simulink model "Copy_of_AB_Final_of_MPC_Bandwidth_Result"  (R2022b)
settings: Solver=FixedStepDiscrete  StartTime=0.0  StopTime=Inf  FixedStep=100e-6  RelTol=1e-3  EnableMultiTasking=on
undefined symbols (not defined in the file): C28x, CPU1, CPU2, CurrentBypassValue, DiscIntNeverNeededParam, Down, GPTRIP1SEL, TZ1, Up
libraries: c2802xlib x31, simulink x22, dspstat3 x17, dspsigops x9, c2837xDlib x6, c280xlib x5, PID_Lib x2, c2000lib x1, spsAlphaBetaZerotoabcLib x1, spsAlphaBetaZerotodq0Lib x1
(part 2 of 8)

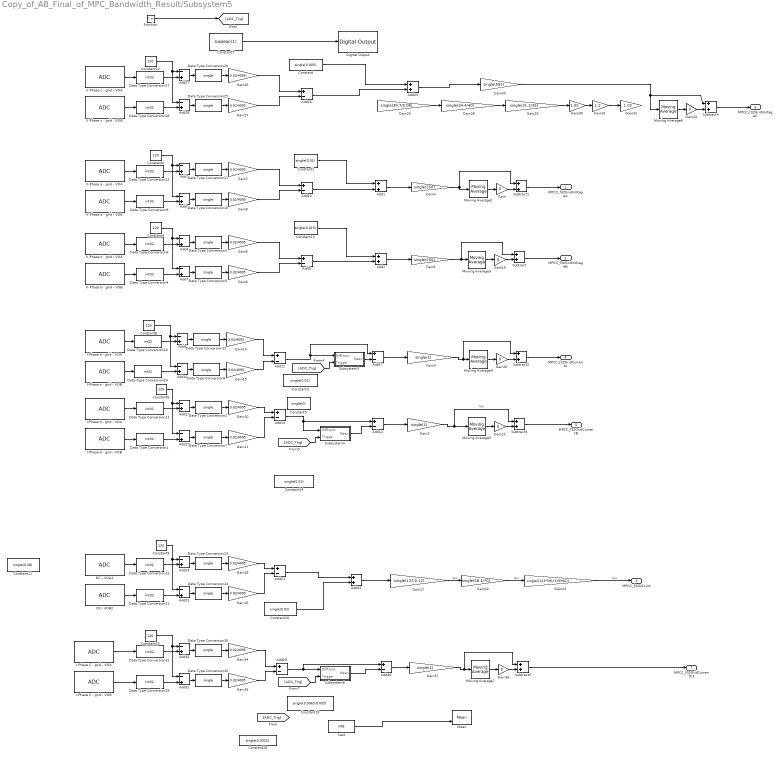
== system Copy_of_AB_Final_of_MPC_Bandwidth_Result/Subsystem5 ==
  function : TriggerPort  TriggerType=function-call  VariantControl=(inherit)  ShowOutputPort=on  OutputDataType=int8
  Add{1..2,22,25} (4 alike) : Sum  AccumDataTypeStr=single  OutDataTypeStr=single
  Add{5,10,12..14,17,21,26,29..30} (10 alike) : Sum  Inputs=+-  AccumDataTypeStr=single  OutDataTypeStr=single
  Add{3..4,6..7,9,11,15,18,23..24,27..28,31..32} (14 alike) : Sum  Inputs=-+  AccumDataTypeStr=single  OutDataTypeStr=single
  Cast : DataTypeConversion  OutDataTypeStr=int8  SaturateOnIntegerOverflow=off  RndMeth=Floor
  Constant : Constant  Value=single(0.005)
  Constant1 : Constant  Value=single(0.01)
  Constant10 : Constant  Value=single(0.02)
  Constant11 : Constant  Value=single(0.28)
  Constant{2,4,6,8..9,12,15} (7 alike) : Constant  Value=120  OutDataTypeStr=single
  Constant13 : Constant  Value=single(0.015)
  Constant14 : Constant  Value=single(0.01)
  Constant18 : Constant  Value=single(0.0025)
  Constant19 : Constant  Value=single(0.0065-0.005)
  Constant3 : Constant  Value=single(0.01)
  Constant5 : Constant  Value=single(0)
  Constant7 : Constant  Value=boolean(1)
  DC - VOA2 : c2802xlib/ADC  blkParamProc=C2000_Type4  ADCModule=C  samplingMode=Single sample mode  ADCResolution=12-bit (Single-ended input)  useSOC1=SOC0  useSOC2=SOC0_SOC1  SOCAcquisitionWindow=22  SOCTriggerSource=ePWM1_ADCSOCA  SOCInterruptTrigger=No ADCINT  Ts=-1  dType=uint16  postInterrupt=off  interruptSel=ADCINT1  ADCINTContinuous=on  endma=off  chdma=1  conv1=ADCINA0  conv2=ADCINA0 and ADCINB0  conv1_Type4=ADCIN5  conv2_Type4=ADCIN0 and ADCIN1
  DC- VOB2 : c2802xlib/ADC  blkParamProc=C2000_Type4  ADCModule=B  samplingMode=Single sample mode  ADCResolution=12-bit (Single-ended input)  useSOC1=SOC3  useSOC2=SOC0_SOC1  SOCAcquisitionWindow=22  SOCTriggerSource=ePWM1_ADCSOCA  SOCInterruptTrigger=No ADCINT  Ts=-1  dType=uint16  postInterrupt=off  interruptSel=ADCINT2  ADCINTContinuous=on  endma=off  chdma=1  conv1=ADCINA0  conv2=ADCINA0 and ADCINB0  conv1_Type4=ADCIN5  conv2_Type4=ADCIN2 and ADCIN3
  Data Type Conversion{1,4,6,9,12..14,16,21..22,27..29,31} (14 alike) : DataTypeConversion  OutDataTypeStr=int32  ConvertRealWorld=Stored Integer (SI)  SaturateOnIntegerOverflow=off  RndMeth=Floor
  Data Type Conversion{2..3,5,7..8,10..11,15,23..26,30,32} (14 alike) : DataTypeConversion  OutDataTypeStr=single  SaturateOnIntegerOverflow=off  RndMeth=Floor
  Digital Output : c2837xDlib/Digital Output  GPIO_Number=GPIO32~GPIO39  GPIO_Bit0=on  GPIO_BIT0_Toggle=on  GPIO_Bit1=off  GPIO_BIT1_Toggle=off  GPIO_Bit2=off  GPIO_BIT2_Toggle=off  GPIO_Bit3=off  GPIO_BIT3_Toggle=off  GPIO_Bit4=off  GPIO_BIT4_Toggle=off  GPIO_Bit5=off  GPIO_BIT5_Toggle=off  GPIO_Bit6=off  GPIO_BIT6_Toggle=off  GPIO_Bit7=off  GPIO_BIT7_Toggle=off
  Gain{,19..21,24,36} (6 alike) : Gain  Gain=0
  Gain1 : Gain  Gain=single(250)
  Gain{5..7,9..11,14..16,18,26..27,34..35} (14 alike) : Gain  Gain=3.02/4095  ParamDataTypeStr=single  OutDataTypeStr=single
  Gain17 : Gain  Gain=single(137/0.22)
  Gain2 : Gain  Gain=single(1)
  Gain22 : Gain  Gain=single(58.4/70)
  Gain23 : Gain  Gain=single((123*59)/(135*60))
  Gain25 : Gain  Gain=single(30.7/0.06)
  Gain28 : Gain  Gain=single(34.4/40)
  Gain29 : Gain  Gain=single(31.2/35)
  Gain3 : Gain  Gain=single(1)
  Gain30 : Gain  Gain=1.05
  Gain31 : Gain  Gain=1.2
  Gain32 : Gain  Gain=1.02
  Gain33 : Gain  Gain=single(505)
  Gain37 : Gain  Gain=single(1)
  Gain4 : Gain  Gain=single(250)
  I-Phase C - grid - VOA : c2802xlib/ADC  blkParamProc=C2000_Type4  ADCModule=A  samplingMode=Single sample mode  ADCResolution=12-bit (Single-ended input)  useSOC1=SOC15  useSOC2=SOC0_SOC1  SOCAcquisitionWindow=22  SOCTriggerSource=ePWM1_ADCSOCA  SOCInterruptTrigger=No ADCINT  Ts=-1  dType=uint16  postInterrupt=off  interruptSel=ADCINT1  ADCINTContinuous=on  endma=off  chdma=1  conv1=ADCINA0  conv2=ADCINA0 and ADCINB0  conv1_Type4=ADCIN15  conv2_Type4=ADCIN0 and ADCIN1
  I-Phase C - grid - VOB : c2802xlib/ADC  blkParamProc=C2000_Type4  ADCModule=A  samplingMode=Single sample mode  ADCResolution=12-bit (Single-ended input)  useSOC1=SOC10  useSOC2=SOC0_SOC1  SOCAcquisitionWindow=22  SOCTriggerSource=ePWM1_ADCSOCA  SOCInterruptTrigger=No ADCINT  Ts=-1  dType=uint16  postInterrupt=off  interruptSel=ADCINT2  ADCINTContinuous=on  endma=off  chdma=1  conv1=ADCINA0  conv2=ADCINA0 and ADCINB0  conv1_Type4=ADCIN14  conv2_Type4=ADCIN2 and ADCIN3
  I-Phase a - grid - VOA : c2802xlib/ADC  blkParamProc=C2000_Type4  ADCModule=A  samplingMode=Single sample mode  ADCResolution=12-bit (Single-ended input)  useSOC1=SOC0  useSOC2=SOC0_SOC1  SOCAcquisitionWindow=22  SOCTriggerSource=ePWM1_ADCSOCA  SOCInterruptTrigger=No ADCINT  Ts=-1  dType=uint16  postInterrupt=on  interruptSel=ADCINT1  ADCINTContinuous=on  endma=off  chdma=1  conv1=ADCINA0  conv2=ADCINA0 and ADCINB0  conv1_Type4=ADCIN4  conv2_Type4=ADCIN0 and ADCIN1
  I-Phase a - grid - VOB : c2802xlib/ADC  blkParamProc=C2000_Type4  ADCModule=B  samplingMode=Single sample mode  ADCResolution=12-bit (Single-ended input)  useSOC1=SOC1  useSOC2=SOC0_SOC1  SOCAcquisitionWindow=22  SOCTriggerSource=ePWM1_ADCSOCA  SOCInterruptTrigger=No ADCINT  Ts=-1  dType=uint16  postInterrupt=off  interruptSel=ADCINT2  ADCINTContinuous=on  endma=off  chdma=1  conv1=ADCINA0  conv2=ADCINA0 and ADCINB0  conv1_Type4=ADCIN4  conv2_Type4=ADCIN2 and ADCIN3
  I-Phase b - grid - VOA : c2802xlib/ADC  blkParamProc=C2000_Type4  ADCModule=C  samplingMode=Single sample mode  ADCResolution=12-bit (Single-ended input)  useSOC1=SOC12  useSOC2=SOC0_SOC1  SOCAcquisitionWindow=22  SOCTriggerSource=ePWM1_ADCSOCA  SOCInterruptTrigger=No ADCINT  Ts=-1  dType=uint16  postInterrupt=off  interruptSel=ADCINT1  ADCINTContinuous=on  endma=off  chdma=1  conv1=ADCINA0  conv2=ADCINA0 and ADCINB0  conv1_Type4=ADCIN4  conv2_Type4=ADCIN0 and ADCIN1
  I-Phase b - grid - VOB : c2802xlib/ADC  blkParamProc=C2000_Type4  ADCModule=A  samplingMode=Single sample mode  ADCResolution=12-bit (Single-ended input)  useSOC1=SOC3  useSOC2=SOC0_SOC1  SOCAcquisitionWindow=22  SOCTriggerSource=ePWM1_ADCSOCA  SOCInterruptTrigger=No ADCINT  Ts=-1  dType=uint16  postInterrupt=off  interruptSel=ADCINT2  ADCINTContinuous=on  endma=off  chdma=1  conv1=ADCINA0  conv2=ADCINA0 and ADCINB0  conv1_Type4=ADCIN5  conv2_Type4=ADCIN2 and ADCIN3
  Mean : dspstat3/Mean  run=on  InputProcessing=Columns as channels (frame based)  reset_popup=Rising edge  directionMode=Each column  dimension=1  roiEnable=off  roiType=Rectangles  roiPortion=Entire ROI  roiOutput=Individual statistics for each ROI  roiFlag=off  roundingMode=Floor  overflowMode=off  outputDataTypeStr=Inherit: Same as accumulator  outputMin=[]  outputMax=[]  outputLastDataTypeStr=Inherit: Same as accumulator
  Moving Average{1,3..7} (6 alike) : dspstat3/Moving Average  Method=Exponential weighting  ForgettingFactorPort=off  SpecifyWindowLength=on  WindowLength=4  OverlapLength=3  AllowArbitraryInputLength=off  ForgettingFactor=0.99  SimulateUsing=Code generation
  Subsystem3 : Subsystem
  Subsystem4 : Subsystem
  Subsystem6 : Subsystem
  Subtract{,1..5} (6 alike) : Sum
  V-Phase a - grid - VOA : c2802xlib/ADC  blkParamProc=C2000_Type4  ADCModule=C  samplingMode=Single sample mode  ADCResolution=12-bit (Single-ended input)  useSOC1=SOC4  useSOC2=SOC0_SOC1  SOCAcquisitionWindow=22  SOCTriggerSource=ePWM1_ADCSOCA  SOCInterruptTrigger=No ADCINT  Ts=-1  dType=uint16  postInterrupt=off  interruptSel=ADCINT1  ADCINTContinuous=on  endma=off  chdma=1  conv1=ADCINA0  conv2=ADCINA0 and ADCINB0  conv1_Type4=ADCIN3  conv2_Type4=ADCIN0 and ADCIN1
  V-Phase a - grid - VOB : c2802xlib/ADC  blkParamProc=C2000_Type4  ADCModule=B  samplingMode=Single sample mode  ADCResolution=12-bit (Single-ended input)  useSOC1=SOC5  useSOC2=SOC0_SOC1  SOCAcquisitionWindow=22  SOCTriggerSource=ePWM1_ADCSOCA  SOCInterruptTrigger=No ADCINT  Ts=-1  dType=uint16  postInterrupt=off  interruptSel=ADCINT2  ADCINTContinuous=on  endma=off  chdma=1  conv1=ADCINA0  conv2=ADCINA0 and ADCINB0  conv1_Type4=ADCIN3  conv2_Type4=ADCIN2 and ADCIN3
  V-Phase b - grid - VOA : c2802xlib/ADC  blkParamProc=C2000_Type4  ADCModule=A  samplingMode=Single sample mode  ADCResolution=12-bit (Single-ended input)  useSOC1=SOC6  useSOC2=SOC0_SOC1  SOCAcquisitionWindow=22  SOCTriggerSource=ePWM1_ADCSOCA  SOCInterruptTrigger=No ADCINT  Ts=-1  dType=uint16  postInterrupt=off  interruptSel=ADCINT1  ADCINTContinuous=on  endma=off  chdma=1  conv1=ADCINA0  conv2=ADCINA0 and ADCINB0  conv1_Type4=ADCIN3  conv2_Type4=ADCIN0 and ADCIN1
  V-Phase b - grid - VOB : c2802xlib/ADC  blkParamProc=C2000_Type4  ADCModule=C  samplingMode=Single sample mode  ADCResolution=12-bit (Single-ended input)  useSOC1=SOC7  useSOC2=SOC0_SOC1  SOCAcquisitionWindow=22  SOCTriggerSource=ePWM1_ADCSOCA  SOCInterruptTrigger=No ADCINT  Ts=-1  dType=uint16  postInterrupt=off  interruptSel=ADCINT2  ADCINTContinuous=on  endma=off  chdma=1  conv1=ADCINA0  conv2=ADCINA0 and ADCINB0  conv1_Type4=ADCIN2  conv2_Type4=ADCIN2 and ADCIN3
  V-Phase c - grid - VOA : c2802xlib/ADC  blkParamProc=C2000_Type4  ADCModule=B  samplingMode=Single sample mode  ADCResolution=12-bit (Single-ended input)  useSOC1=SOC0  useSOC2=SOC0_SOC1  SOCAcquisitionWindow=22  SOCTriggerSource=ePWM1_ADCSOCA  SOCInterruptTrigger=No ADCINT  Ts=-1  dType=uint16  postInterrupt=off  interruptSel=ADCINT1  ADCINTContinuous=on  endma=off  chdma=1  conv1=ADCINA0  conv2=ADCINA0 and ADCINB0  conv1_Type4=ADCIN2  conv2_Type4=ADCIN0 and ADCIN1
  V-Phase c - grid - VOB : c2802xlib/ADC  blkParamProc=C2000_Type4  ADCModule=A  samplingMode=Single sample mode  ADCResolution=12-bit (Single-ended input)  useSOC1=SOC1  useSOC2=SOC0_SOC1  SOCAcquisitionWindow=22  SOCTriggerSource=ePWM1_ADCSOCA  SOCInterruptTrigger=No ADCINT  Ts=-1  dType=uint16  postInterrupt=off  interruptSel=ADCINT2  ADCINTContinuous=on  endma=off  chdma=1  conv1=ADCINA0  conv2=ADCINA0 and ADCINB0  conv1_Type4=ADCIN2  conv2_Type4=ADCIN2 and ADCIN3
  MPCC_f32GridVoltageA : Outport
  MPCC_f32GridVoltageB : Outport  Port=2
  MPCC_f32DCLink : Outport  Port=3
  MPCC_f32GridCurrentA : Outport  Port=4
  MPCC_f32GridCurrentB : Outport  Port=5
  MPCC_f32GridVoltageC : Outport  Port=6
  MPCC_f32GridCurrentC3 : Outport  Port=7
  wires:
  Gain5/1 -> Add5/1
  Data Type Conversion5/1 -> Gain5/1
  Gain1/1 -> Subtract/1, Moving Average3/1
  Add9/1 -> Data Type Conversion10/1
  V-Phase a - grid - VOB/1 -> Data Type Conversion9/1
  Data Type Conversion9/1 -> Add9/2
  Gain7/1 -> Add10/1
  Data Type Conversion10/1 -> Gain9/1
  Data Type Conversion12/1 -> Add3/2
  Add7/1 -> Data Type Conversion3/1
  Data Type Conversion4/1 -> Add7/2
  Data Type Conversion6/1 -> Add4/2
  Gain9/1 -> Add10/2
  V-Phase b - grid - VOB/1 -> Data Type Conversion4/1
  V-Phase b - grid - VOA/1 -> Data Type Conversion6/1
  Add4/1 -> Data Type Conversion5/1
  Add3/1 -> Data Type Conversion11/1
  Data Type Conversion3/1 -> Gain6/1
  Gain6/1 -> Add5/2
  Constant4/1 -> Add7/1, Add4/1
  V-Phase a - grid - VOA/1 -> Data Type Conversion12/1
  Constant2/1 -> Add9/1, Add3/1
  Data Type Conversion11/1 -> Gain7/1
  Add1/1 -> Gain4/1
  Add2/1 -> Gain1/1
  I-Phase b - grid - VOA/1 -> Data Type Conversion13/1
  Data Type Conversion15/1 -> Gain14/1
  Data Type Conversion8/1 -> Gain15/1
  Data Type Conversion14/1 -> Add18/2
  Gain15/1 -> Add12/2
  Data Type Conversion13/1 -> Add11/2
  Data Type Conversion16/1 -> Add6/2
  Gain14/1 -> Add12/1
  Add6/1 -> Data Type Conversion15/1
  Gain10/1 -> Add13/1
  Add18/1 -> Data Type Conversion8/1
  I-Phase a - grid - VOA/1 -> Data Type Conversion16/1
  Gain2/1 -> Subtract3/1, Moving Average5/1  "Iau"
  Data Type Conversion2/1 -> Gain10/1
  Constant6/1 -> Add15/1, Add11/1
  I-Phase b - grid - VOB/1 -> Data Type Conversion1/1
  Data Type Conversion1/1 -> Add15/2
  Gain11/1 -> Add13/2
  Add17/1 -> Gain3/1
  Add11/1 -> Data Type Conversion2/1
  Constant8/1 -> Add18/1, Add6/1
  I-Phase a - grid - VOB/1 -> Data Type Conversion14/1
  Data Type Conversion7/1 -> Gain11/1
  Add15/1 -> Data Type Conversion7/1
  Subtract/1 -> MPCC_f32GridVoltageB/1
  Moving Average3/1 -> Gain19/1
  Moving Average1/1 -> Gain/1
  Gain4/1 -> Subtract1/1, Moving Average1/1
  Subtract1/1 -> MPCC_f32GridVoltageA/1
  Moving Average4/1 -> Gain20/1
  Gain3/1 -> Subtract2/1, Moving Average4/1
  Moving Average5/1 -> Gain21/1
  Data Type Conversion22/1 -> Add24/2
  DC- VOB2/1 -> Data Type Conversion21/1
  Data Type Conversion21/1 -> Add23/2
  Data Type Conversion23/1 -> Gain18/1
  DC - VOA2/1 -> Data Type Conversion22/1
  Add24/1 -> Data Type Conversion23/1
  Constant9/1 -> Add23/1, Add24/1
  Gain16/1 -> Add21/2
  Add23/1 -> Data Type Conversion24/1
  Data Type Conversion24/1 -> Gain16/1
  Gain18/1 -> Add21/1
  Gain/1 -> Subtract1/2
  Gain19/1 -> Subtract/2
  Gain20/1 -> Subtract2/2
  Gain21/1 -> Subtract3/2
  Gain17/1 -> Gain22/1  "Iau"
  Subtract2/1 -> MPCC_f32GridCurrentA/1
  Subtract3/1 -> MPCC_f32GridCurrentB/1
  Gain22/1 -> Gain23/1  "Iau"
  V-Phase c - grid - VOB/1 -> Data Type Conversion28/1
  Gain26/1 -> Add26/1
  Data Type Conversion25/1 -> Gain27/1
  V-Phase c - grid - VOA/1 -> Data Type Conversion27/1
  Subtract4/1 -> MPCC_f32GridVoltageC/1
  Data Type Conversion26/1 -> Gain26/1
  Data Type Conversion27/1 -> Add27/2
  Moving Average6/1 -> Gain24/1
  Data Type Conversion28/1 -> Add28/2
  Gain27/1 -> Add26/2
  Add28/1 -> Data Type Conversion25/1
  Constant12/1 -> Add28/1, Add27/1
  Add27/1 -> Data Type Conversion26/1
  Gain25/1 -> Gain28/1
  Gain24/1 -> Subtract4/2
  Gain28/1 -> Gain29/1
  Gain29/1 -> Gain30/1
  Gain30/1 -> Gain31/1
  Gain31/1 -> Gain32/1
  Gain33/1 -> Subtract4/1, Moving Average6/1
  Add31/1 -> Data Type Conversion32/1
  Data Type Conversion32/1 -> Gain35/1
  Data Type Conversion31/1 -> Add32/2
  Gain34/1 -> Add29/1
  Constant15/1 -> Add31/1, Add32/1
  Gain35/1 -> Add29/2
  Subtract5/1 -> MPCC_f32GridCurrentC3/1
  Gain36/1 -> Subtract5/2
  Data Type Conversion30/1 -> Gain34/1
  Data Type Conversion29/1 -> Add31/2
  I-Phase C - grid - VOB/1 -> Data Type Conversion29/1
  I-Phase C - grid - VOA/1 -> Data Type Conversion31/1
  Gain37/1 -> Subtract5/1, Moving Average7/1
  Add32/1 -> Data Type Conversion30/1
  Add30/1 -> Gain37/1
  Moving Average7/1 -> Gain36/1
  Add22/1 -> Gain17/1
  Constant7/1 -> Digital Output/1
  Add14/1 -> Gain2/1
  function/1 -> [ADC_Trig]
  Cast/1 -> Mean/2
  Add25/1 -> Gain33/1
  [ADC_Trig] -> Subsystem3/2(Trigger)
  Add12/1 -> Add17/1, Subsystem3/1(DiffInput)
  Subsystem3/1(Mean) -> Add17/2
  [ADC_Trig] -> Subsystem4/2(Trigger)
  Add13/1 -> Add14/1, Subsystem4/1(DiffInput)
  Subsystem4/1(Mean) -> Add14/2
  [ADC_Trig] -> Subsystem6/2(Trigger)
  Add29/1 -> Add30/1, Subsystem6/1(DiffInput)
  Subsystem6/1(Mean) -> Add30/2
  Constant/1 -> Add25/1
  Add26/1 -> Add25/2
  Constant1/1 -> Add1/1
  Add10/1 -> Add1/2
  Constant13/1 -> Add2/1
  Add5/1 -> Add2/2
  Gain23/1 -> MPCC_f32DCLink/1  "Iau"
  Add21/1 -> Add22/1
  Constant10/1 -> Add22/2

== system Copy_of_AB_Final_of_MPC_Bandwidth_Result/Voltage_Loop ==
  PI_f32DCLinkVoltageRef : Inport
  PI_f32DCLinkVoltage : Inport  Port=2
  PI_f32DCLink : Inport  Port=3
  VoltageLoop_FC : TriggerPort  TriggerType=function-call  VariantControl=(inherit)  SampleTime=-1
      settings: AttributesFormatString=|
      | %<StatesWhenEnabling>
      | %<SampleTime>
  Add : Sum  Inputs=+-
  Cast To Single : DataTypeConversion  OutDataTypeStr=single  SaturateOnIntegerOverflow=off  RndMeth=Floor
  Cast To Single1 : DataTypeConversion  OutDataTypeStr=single  SaturateOnIntegerOverflow=off  RndMeth=Floor
  Cast To Single3 : DataTypeConversion  OutDataTypeStr=single  SaturateOnIntegerOverflow=off  RndMeth=Floor
  Constant : Constant  Commented=on  Value=single(0.2)
  Constant1 : Constant  Commented=on  Value=single(10)
  Constant10 : Constant  Value=single(2.5)
  Constant11 : Constant  Value=single(0.1)
  Constant12 : Constant  Value=single(0.8685252)
  Constant13 : Constant  Value=single(0.01955)
  Constant2 : Constant  Value=single(7/7)
  Constant3 : Constant  Value=boolean(1)
  Constant4 : Constant  Value=boolean(0)
  Constant5 : Constant  Value=boolean(1)
  Constant6 : Constant  Value=single(0.2)
  Constant7 : Constant  Value=single(0)
  Constant8 : Constant  Commented=on  Value=CurrentBypassValue
  Constant9 : Constant  Value=single(10)
  Gain : Gain  Gain=-1
  Gain1 : Gain  Gain=single(7)
  Gain2 : Gain  Gain=1/300
  Gain3 : Gain  Gain=1/300
  Mux2 : Mux  Inputs=3
  PI : PID_Lib/PI  SystemSampleTime=-1  VariantActivationTime=update diagram  Latency=0  AutoFrameSizeCalculation=off
  Scope : Scope
  Step : Step  Time=30  Before=-0.5  After=-1.5
  Step1 : Step  Time=30  Before=200  After=300
  Subsystem5 : Subsystem  Commented=through
  Switch : Switch  Criteria=u2 ~= 0  SaturateOnIntegerOverflow=off  InputSameDT=off
  Terminator{,1..4} (5 alike) : Terminator
  PI_f32DGridCurrentReference : Outport
  MPCC_f32DCLinkFiltered : Outport  Port=2
  MPCC_f32DCLinkref : Outport  Port=3
  wires:
  Constant2/1 -> Gain/1, PI/4
  Gain/1 -> PI/5
  Constant3/1 -> PI/6
  Constant4/1 -> PI/7
  PI/2 -> Terminator/1
  PI/3 -> Terminator1/1
  PI/4 -> Terminator2/1
  PI/5 -> Terminator3/1
  Constant5/1 -> Switch/2
  PI/1 -> Switch/1, Scope/1
  Switch/1 -> Cast To Single/1
  Cast To Single1/1 -> Gain2/1
  Cast To Single/1 -> Gain1/1
  Cast To Single3/1 -> Gain3/1, MPCC_f32DCLinkref/1
  PI_f32DCLinkVoltage/1 -> Subsystem5/1(MPCC_f32DCLink)
  Subsystem5/1(MPCC_f32DCLinkFiltered) -> MPCC_f32DCLinkFiltered/1, Cast To Single1/1
  Constant7/1 -> PI/8
  Step/1 -> Switch/3
  Add/1 -> Mux2/1, PI/1
  Gain1/1 -> Mux2/2, PI_f32DGridCurrentReference/1
  Gain3/1 -> Add/1
  Gain2/1 -> Add/2
  PI_f32DCLink/1 -> Mux2/3
  Mux2/1 -> Terminator4/1
  PI_f32DCLinkVoltageRef/1 -> Cast To Single3/1
  Constant6/1 -> PI/2
  Constant9/1 -> PI/3

== system Copy_of_AB_Final_of_MPC_Bandwidth_Result/Subsystem1/ABCtoDQO ==
  PI_f32GridCurrentA : Inport
  PI_f32GridCurrentB : Inport  Port=2
  PI_f32GridCurrentC : Inport  Port=3
  PI_f32GridVoltageA : Inport  Port=4
  PI_f32GridVoltageB : Inport  Port=5
  PI_f32GridVoltageC : Inport  Port=6
  PI_f32ElectricalAngle : Inport  Port=7
  MPCC_f32AngularFrequency : Inport  Port=8
  ABCtoDQOCurrent : Subsystem  Commented=on
  ABCtoDQOVoltage : Subsystem  Commented=on
  Cast To Single : DataTypeConversion  OutDataTypeStr=single  SaturateOnIntegerOverflow=off  RndMeth=Floor
  Cast To Single1 : DataTypeConversion  OutDataTypeStr=single  SaturateOnIntegerOverflow=off  RndMeth=Floor
  Constant : Constant
  Gain1 : Gain  Gain=single(100e-6)
  Ground : Ground
  abc_dq : Subsystem
  abc_dq1 : Subsystem
  abc_dq4 : Subsystem
  PI_f32DGridCurrent : Outport
  PI_f32QGridCurrent : Outport  Port=2
  PI_f32OGridCurrent : Outport  Port=3
  PI_f32DGridVoltage : Outport  Port=4
  PI_f32QGridVoltage : Outport  Port=5
  PI_f32OGridVoltage : Outport  Port=6
  PI_f32DGridVoltage1 : Outport  Port=7
  PI_f32QGridVoltage1 : Outport  Port=8
  wires:
  abc_dq/1(Id) -> Cast To Single/1
  abc_dq/2(Iq) -> Cast To Single1/1
  PI_f32ElectricalAngle/1 -> [PI_f32ElectricalAngle]
  [PI_f32ElectricalAngle] -> abc_dq/1(theta)
  Ground/1 -> PI_f32OGridCurrent/1, PI_f32OGridVoltage/1
  abc_dq1/2(Iq) -> PI_f32QGridVoltage/1
  [PI_f32ElectricalAngle] -> abc_dq1/1(theta)
  abc_dq1/1(Id) -> PI_f32DGridVoltage/1
  PI_f32GridCurrentC/1 -> abc_dq/4(c)
  PI_f32GridCurrentB/1 -> abc_dq/3(b)
  PI_f32GridCurrentA/1 -> abc_dq/2(a)
  PI_f32GridVoltageA/1 -> abc_dq4/2(a), abc_dq1/2(a)
  PI_f32GridVoltageB/1 -> abc_dq1/3(b), abc_dq4/3(b)
  PI_f32GridVoltageC/1 -> abc_dq1/4(c), abc_dq4/4(c)
  Cast To Single/1 -> PI_f32DGridCurrent/1
  Cast To Single1/1 -> PI_f32QGridCurrent/1
  MPCC_f32AngularFrequency/1 -> [MPCC_f32AngularFrequency]
  Gain1/1 -> abc_dq4/1(theta)
  Constant/1 -> abc_dq4/5(c1)
  [MPCC_f32AngularFrequency] -> Gain1/1
  abc_dq4/1(Id) -> PI_f32DGridVoltage1/1
  abc_dq4/2(Iq) -> PI_f32QGridVoltage1/1

== system Copy_of_AB_Final_of_MPC_Bandwidth_Result/Subsystem1/AlphaBetaDutiesCalculation ==
  MPCC_f32DVoltageReference : Inport
  MPCC_f32QVoltageReference : Inport  Port=2
  MPCC_f32ElectricalAngle_K_1 : Inport  Port=3
  MPCC_f32DCLinkVoltage : Inport  Port=4
  AlphaBetaVoltageReferenceCalculation : Subsystem
  DutiesCalculation : Subsystem
  MPCC_f32AlphaVoltageReference : Outport
  MPCC_f32BetaVoltageReference : Outport  Port=2
  MPCC_f32Duty_Sector1 : Outport  Port=3
  MPCC_f32Duty_Sector2 : Outport  Port=4
  MPCC_f32Duty_Sector3 : Outport  Port=5
  MPCC_f32Duty_Sector4 : Outport  Port=6
  MPCC_f32Duty_Sector5 : Outport  Port=7
  MPCC_f32Duty_Sector6 : Outport  Port=8
  wires:
  MPCC_f32ElectricalAngle_K_1/1 -> AlphaBetaVoltageReferenceCalculation/3(MPCC_f32ElectricalAngle_K_1)
  AlphaBetaVoltageReferenceCalculation/1(MPCC_f32AlphaVoltageReference) -> MPCC_f32AlphaVoltageReference/1
  AlphaBetaVoltageReferenceCalculation/2(MPCC_f32BetaVoltageReference) -> MPCC_f32BetaVoltageReference/1
  DutiesCalculation/1(MPCC_f32Duty_Sector1) -> MPCC_f32Duty_Sector1/1
  DutiesCalculation/2(MPCC_f32Duty_Sector2) -> MPCC_f32Duty_Sector2/1
  DutiesCalculation/3(MPCC_f32Duty_Sector3) -> MPCC_f32Duty_Sector3/1
  DutiesCalculation/4(MPCC_f32Duty_Sector4) -> MPCC_f32Duty_Sector4/1
  DutiesCalculation/6(MPCC_f32Duty_Sector6) -> MPCC_f32Duty_Sector6/1
  DutiesCalculation/5(MPCC_f32Duty_Sector5) -> MPCC_f32Duty_Sector5/1
  MPCC_f32DCLinkVoltage/1 -> DutiesCalculation/3(MPCC_f32DCLinkVoltage)
  [MPCC_f32AlphaVoltageReference] -> DutiesCalculation/1(MPCC_f32AlphaVoltageReference)
  [MPCC_f32BetaVoltageReference] -> DutiesCalculation/2(MPCC_f32BetaVoltageReference)
  MPCC_f32DVoltageReference/1 -> [MPCC_f32AlphaVoltageReference]
  MPCC_f32QVoltageReference/1 -> [MPCC_f32BetaVoltageReference]

== system Copy_of_AB_Final_of_MPC_Bandwidth_Result/Subsystem1/AlphaBetaVoltageReferenceCalculation ==
  MPCC_f32DVoltageReference : Inport
  MPCC_f32QVoltageReference : Inport  Port=2
  MPCC_f32ElectricalAngle_K_1 : Inport  Port=3
  Add : Sum  Inputs=+-
  Add1 : Sum
  Product{,1..3} (4 alike) : Product
  Sin : Trigonometry  Operator=cos
  Sin1 : Trigonometry
  Sin2 : Trigonometry
  Sin3 : Trigonometry  Operator=cos
  MPCC_f32AlphaVoltageReference : Outport
  MPCC_f32BetaVoltageReference : Outport  Port=2
  wires:
  Sin2/1 -> Product2/1
  [MPCC_f32QVoltageReference] -> Product3/2
  Sin1/1 -> Product1/1
  Sin3/1 -> Product3/1
  Product/1 -> Add/1
  [MPCC_f32DVoltageReference] -> Product2/2
  [MPCC_f32ElectricalAngle_K_1] -> Sin2/1
  [MPCC_f32QVoltageReference] -> Product1/2
  Add1/1 -> MPCC_f32BetaVoltageReference/1
  Product2/1 -> Add1/1
  Product3/1 -> Add1/2
  [MPCC_f32ElectricalAngle_K_1] -> Sin3/1
  MPCC_f32DVoltageReference/1 -> [MPCC_f32DVoltageReference]
  Add/1 -> MPCC_f32AlphaVoltageReference/1
  [MPCC_f32ElectricalAngle_K_1] -> Sin/1
  [MPCC_f32DVoltageReference] -> Product/2
  MPCC_f32QVoltageReference/1 -> [MPCC_f32QVoltageReference]
  Product1/1 -> Add/2
  Sin/1 -> Product/1
  [MPCC_f32ElectricalAngle_K_1] -> Sin1/1
  MPCC_f32ElectricalAngle_K_1/1 -> [MPCC_f32ElectricalAngle_K_1]

== system Copy_of_AB_Final_of_MPC_Bandwidth_Result/Subsystem1/CodeGeneration ==
  Input : Inport
  Add : Sum  Inputs=+-  OutDataTypeStr=Inherit: Same as first input
  Demux2 : Demux  Outputs=2
  Index Vector : MultiPortSwitch  Inputs=1  SaturateOnIntegerOverflow=off  InputSameDT=off
  SCI Transmit : c280xlib/SCI Transmit  sciModule=A  dataHead=''  dataTail=''  blockingMode=on  outputStatus=off
  While Iterator : WhileIterator  MaxIters=-1  WhileBlockType=do-while  ShowIterationPort=on  OutputDataType=int16
  wires:
  While Iterator/1 -> Add/2, Index Vector/1
  Demux2/1 -> Index Vector/2
  Index Vector/1 -> SCI Transmit/1
  Add/1 -> While Iterator/1
  Demux2/2 -> Add/1
  Input/1 -> Demux2/1

== system Copy_of_AB_Final_of_MPC_Bandwidth_Result/Subsystem1/CodeGeneration1 ==
  Input : Inport
  Add : Sum  Inputs=+-  OutDataTypeStr=Inherit: Same as first input
  Demux2 : Demux  Outputs=2
  Index Vector : MultiPortSwitch  Inputs=1  SaturateOnIntegerOverflow=off  InputSameDT=off
  SCI Transmit : c280xlib/SCI Transmit  sciModule=A  dataHead=''  dataTail=''  blockingMode=on  outputStatus=off
  While Iterator : WhileIterator  MaxIters=-1  WhileBlockType=do-while  ShowIterationPort=on  OutputDataType=int16
  wires:
  While Iterator/1 -> Add/2, Index Vector/1
  Demux2/1 -> Index Vector/2
  Index Vector/1 -> SCI Transmit/1
  Add/1 -> While Iterator/1
  Demux2/2 -> Add/1
  Input/1 -> Demux2/1

== system Copy_of_AB_Final_of_MPC_Bandwidth_Result/Subsystem1/Data ==
  Data : Inport
  Data_width : Inport  Port=2
  Action Port : ActionPort  ActionPortLabel=else
  Mux : Mux  Inputs=2
  Start : Constant  Value=hex2dec('0000')  OutDataTypeStr=uint16
  Data_out : Outport  VectorParamsAs1DForOutWhenUnconnected=off
  Iteration : Outport  Port=2  VectorParamsAs1DForOutWhenUnconnected=off
  wires:
  Start/1 -> Mux/2
  Mux/1 -> Data_out/1
  Data/1 -> Mux/1
  Data_width/1 -> Iteration/1

== system Copy_of_AB_Final_of_MPC_Bandwidth_Result/Subsystem1/Data1 ==
  Data : Inport
  Data_width : Inport  Port=2
  Action Port : ActionPort  ActionPortLabel=else
  Mux : Mux  Inputs=2
  Start : Constant  Value=hex2dec('0000')  OutDataTypeStr=uint16
  Data_out : Outport  VectorParamsAs1DForOutWhenUnconnected=off
  Iteration : Outport  Port=2  VectorParamsAs1DForOutWhenUnconnected=off
  wires:
  Start/1 -> Mux/2
  Mux/1 -> Data_out/1
  Data/1 -> Mux/1
  Data_width/1 -> Iteration/1

== system Copy_of_AB_Final_of_MPC_Bandwidth_Result/Subsystem1/Data_Conditioning ==
  In1 : Inport
  Data Type Conversion3 : DataTypeConversion  OutDataTypeStr=uint16  ConvertRealWorld=Stored Integer (SI)  SaturateOnIntegerOverflow=off  RndMeth=Floor
  Out1 : Outport  VectorParamsAs1DForOutWhenUnconnected=off
  wires:
  Data Type Conversion3/1 -> Out1/1
  In1/1 -> Data Type Conversion3/1

== system Copy_of_AB_Final_of_MPC_Bandwidth_Result/Subsystem1/Data_Conditioning1 ==
  In1 : Inport
  Data Type Conversion3 : DataTypeConversion  OutDataTypeStr=uint16  ConvertRealWorld=Stored Integer (SI)  SaturateOnIntegerOverflow=off  RndMeth=Floor
  Out1 : Outport  VectorParamsAs1DForOutWhenUnconnected=off
  wires:
  Data Type Conversion3/1 -> Out1/1
  In1/1 -> Data Type Conversion3/1

== system Copy_of_AB_Final_of_MPC_Bandwidth_Result/Subsystem1/End ==
  Data : Inport
  Data_width : Inport  Port=2
  Action Port : ActionPort  ActionPortLabel=elseif(u1 == 599)
  Bias : Bias  Bias=1  SaturateOnIntegerOverflow=off
  Mux : Mux  Inputs=2
  Start : Constant  Value=hex2dec('4545')  OutDataTypeStr=uint16
  Data_out : Outport  VectorParamsAs1DForOutWhenUnconnected=off
  Iteration : Outport  Port=2  VectorParamsAs1DForOutWhenUnconnected=off
  wires:
  Mux/1 -> Data_out/1
  Data_width/1 -> Bias/1
  Start/1 -> Mux/2
  Bias/1 -> Iteration/1
  Data/1 -> Mux/1

== system Copy_of_AB_Final_of_MPC_Bandwidth_Result/Subsystem1/End1 ==
  Data : Inport
  Data_width : Inport  Port=2
  Action Port : ActionPort  ActionPortLabel=elseif(u1 == 599)
  Bias : Bias  Bias=1  SaturateOnIntegerOverflow=off
  Mux : Mux  Inputs=2
  Start : Constant  Value=hex2dec('4545')  OutDataTypeStr=uint16
  Data_out : Outport  VectorParamsAs1DForOutWhenUnconnected=off
  Iteration : Outport  Port=2  VectorParamsAs1DForOutWhenUnconnected=off
  wires:
  Mux/1 -> Data_out/1
  Data_width/1 -> Bias/1
  Start/1 -> Mux/2
  Bias/1 -> Iteration/1
  Data/1 -> Mux/1

== system Copy_of_AB_Final_of_MPC_Bandwidth_Result/Subsystem1/GridCurrentFirstPrediction ==
  MPCC_f32Predictionterm_A : Inport
  MPCC_f32Predictionterm_B : Inport  Port=2
  MPCC_f32Predictionterm_C : Inport  Port=3
  MPCC_f32DGridCurrent : Inport  Port=4
  MPCC_f32QGridCurrent : Inport  Port=5
  MPCC_f32DGridVoltage : Inport  Port=6
  MPCC_f32QGridVoltage : Inport  Port=7
  MPCC_f32DConvVoltage : Inport  Port=8
  MPCC_f32QConvVoltage : Inport  Port=9
  PredictedIdGridCurrentCalculation : Subsystem
  PredictedIqGridCurrentCalculation : Subsystem
  MPCC_f32DGridCurrent_K_1 : Outport
  MPCC_f32QGridCurrent_K_1 : Outport  Port=2
  wires:
  MPCC_f32DGridVoltage/1 -> [MPCC_f32DGridVoltage]
  MPCC_f32Predictionterm_A/1 -> [MPCC_f32Predictionterm_A]
  MPCC_f32QGridVoltage/1 -> [MPCC_f32QGridVoltage]
  MPCC_f32Predictionterm_C/1 -> [MPCC_f32Predictionterm_C]
  MPCC_f32Predictionterm_B/1 -> [MPCC_f32Predictionterm_B]
  MPCC_f32DGridCurrent/1 -> [MPCC_f32DGridCurrent]
  MPCC_f32QGridCurrent/1 -> [MPCC_f32QGridCurrent]
  PredictedIdGridCurrentCalculation/1(MPCC_f32DGridCurrent_K_1) -> MPCC_f32DGridCurrent_K_1/1
  PredictedIqGridCurrentCalculation/1(MPCC_f32QVoltageReference) -> MPCC_f32QGridCurrent_K_1/1
  [MPCC_f32Predictionterm_A] -> PredictedIdGridCurrentCalculation/1(MPCC_f32Predictionterm_A)
  [MPCC_f32Predictionterm_B] -> PredictedIdGridCurrentCalculation/2(MPCC_f32Predictionterm_B)
  [MPCC_f32Predictionterm_C] -> PredictedIdGridCurrentCalculation/3(MPCC_f32Predictionterm_C)
  [MPCC_f32DGridCurrent] -> PredictedIdGridCurrentCalculation/4(MPCC_f32DGridCurrent)
  [MPCC_f32QGridCurrent] -> PredictedIdGridCurrentCalculation/5(MPCC_f32QGridCurrent)
  [MPCC_f32DGridVoltage] -> PredictedIdGridCurrentCalculation/6(MPCC_f32DGridVoltage)
  [MPCC_f32DConvVoltage] -> PredictedIdGridCurrentCalculation/7(MPCC_f32DConvVoltage)
  MPCC_f32DConvVoltage/1 -> [MPCC_f32DConvVoltage]
  MPCC_f32QConvVoltage/1 -> [MPCC_f32QConvVoltage]
  [MPCC_f32Predictionterm_A] -> PredictedIqGridCurrentCalculation/1(MPCC_f32Predictionterm_A)
  [MPCC_f32Predictionterm_C] -> PredictedIqGridCurrentCalculation/3(MPCC_f32Predictionterm_C)
  [MPCC_f32QGridCurrent] -> PredictedIqGridCurrentCalculation/5(MPCC_f32QGridCurrent)
  [MPCC_f32QGridVoltage] -> PredictedIqGridCurrentCalculation/6(MPCC_f32QGridVoltage)
  [MPCC_f32QConvVoltage] -> PredictedIqGridCurrentCalculation/7(MPCC_f32QConvVoltage)
  [MPCC_f32Predictionterm_B] -> PredictedIqGridCurrentCalculation/2(MPCC_f32Predictionterm_B)
  [MPCC_f32DGridCurrent] -> PredictedIqGridCurrentCalculation/4(MPCC_f32DGridCurrent)

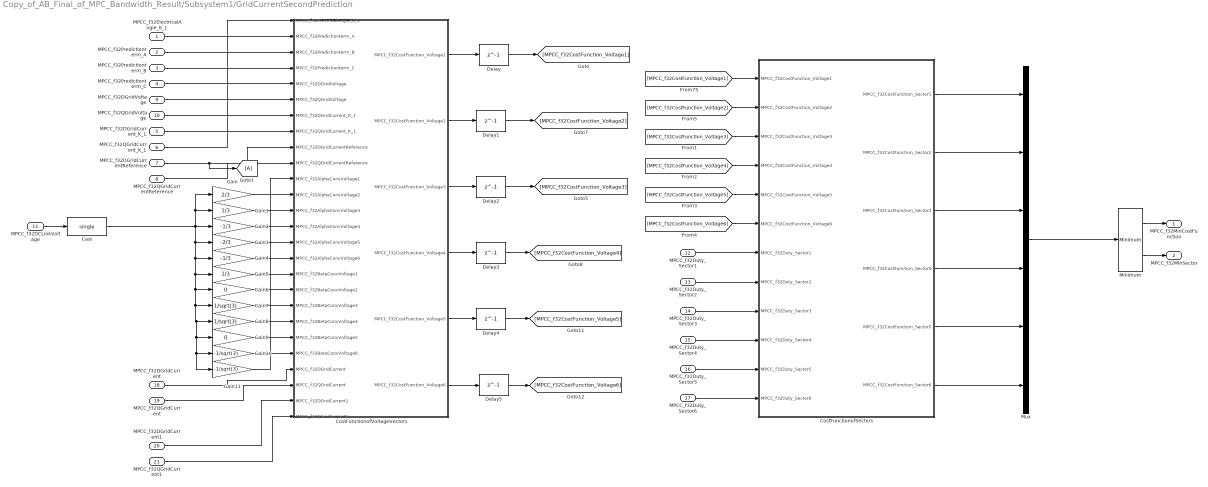
== system Copy_of_AB_Final_of_MPC_Bandwidth_Result/Subsystem1/GridCurrentSecondPrediction ==
  MPCC_f32ElectricalAngle_K_1 : Inport
  MPCC_f32Predictionterm_A : Inport  Port=2
  MPCC_f32Predictionterm_B : Inport  Port=3
  MPCC_f32Predictionterm_C : Inport  Port=4
  MPCC_f32DGridCurrent_K_1 : Inport  Port=5
  MPCC_f32QGridCurrent_K_1 : Inport  Port=6
  MPCC_f32DGridCurrentReference : Inport  Port=7
  MPCC_f32QGridCurrentReference : Inport  Port=8
  MPCC_f32DGridVoltage : Inport  Port=9
  MPCC_f32QGridVoltage : Inport  Port=10
  MPCC_f32DCLinkVoltage : Inport  Port=11
  MPCC_f32Duty_Sector1 : Inport  Port=12
  MPCC_f32Duty_Sector2 : Inport  Port=13
  MPCC_f32Duty_Sector3 : Inport  Port=14
  MPCC_f32Duty_Sector4 : Inport  Port=15
  MPCC_f32Duty_Sector5 : Inport  Port=16
  MPCC_f32Duty_Sector6 : Inport  Port=17
  MPCC_f32DGridCurrent : Inport  Port=18
  MPCC_f32QGridCurrent : Inport  Port=19
  MPCC_f32DGridCurrent1 : Inport  Port=20
  MPCC_f32QGridCurrent1 : Inport  Port=21
  Cast : DataTypeConversion  OutDataTypeStr=single  SaturateOnIntegerOverflow=off  RndMeth=Floor
  CostFunctionofSectors : Subsystem
  CostFunctionofVoltageVectors : Subsystem
  Delay{,1..5} (6 alike) : Delay  DelayLength=1  InitialCondition=single(1000000)  UseCircularBuffer=on
  Gain : Gain  Gain=2/3
  Gain1 : Gain  Gain=1/3
  Gain10 : Gain  Gain=-1/sqrt(3)
  Gain11 : Gain  Gain=-1/sqrt(3)
  Gain2 : Gain  Gain=-1/3
  Gain3 : Gain  Gain=-2/3
  Gain4 : Gain  Gain=-1/3
  Gain5 : Gain  Gain=1/3
  Gain6 : Gain  Gain=0
  Gain7 : Gain  Gain=1/sqrt(3)
  Gain8 : Gain  Gain=1/sqrt(3)
  Gain9 : Gain  Gain=0
  Goto1 : Goto
  Minimum : dspstat3/Minimum  operation=minimum  fcn=Value and Index  indexBase=One  operateOver=Each column  Dimension=1  InputProcessing=Columns as channels (frame based)  reset=None  roiEnable=off  roiType=Rectangles  roiPortion=Entire ROI  roiOutput=Individual statistics for each ROI  roiFlag=off  roundingMode=Floor  overflowMode=off
  Mux : Mux  Inputs=6
  MPCC_f32MinCostFunction : Outport
  MPCC_f32MinSector : Outport  Port=2
  wires:
  CostFunctionofVoltageVectors/3(MPCC_f32CostFunction_Voltage3) -> Delay2/1
  CostFunctionofVoltageVectors/2(MPCC_f32CostFunction_Voltage2) -> Delay1/1
  CostFunctionofVoltageVectors/5(MPCC_f32CostFunction_Voltage5) -> Delay4/1
  CostFunctionofVoltageVectors/6(MPCC_f32CostFunction_Voltage6) -> Delay5/1
  CostFunctionofVoltageVectors/4(MPCC_f32CostFunction_Voltage4) -> Delay3/1
  CostFunctionofVoltageVectors/1(MPCC_f32CostFunction_Voltage1) -> Delay/1
  MPCC_f32ElectricalAngle_K_1/1 -> CostFunctionofVoltageVectors/1(MPCC_f32ElectricalAngle_K_1)
  MPCC_f32Predictionterm_A/1 -> CostFunctionofVoltageVectors/2(MPCC_f32Predictionterm_A)
  MPCC_f32Predictionterm_B/1 -> CostFunctionofVoltageVectors/3(MPCC_f32Predictionterm_B)
  MPCC_f32Predictionterm_C/1 -> CostFunctionofVoltageVectors/4(MPCC_f32Predictionterm_C)
  MPCC_f32DGridVoltage/1 -> CostFunctionofVoltageVectors/5(MPCC_f32DGridVoltage)
  MPCC_f32QGridVoltage/1 -> CostFunctionofVoltageVectors/6(MPCC_f32QGridVoltage)
  MPCC_f32DGridCurrent_K_1/1 -> CostFunctionofVoltageVectors/7(MPCC_f32DGridCurrent_K_1)
  MPCC_f32QGridCurrent_K_1/1 -> CostFunctionofVoltageVectors/8(MPCC_f32QGridCurrent_K_1)
  MPCC_f32DGridCurrentReference/1 -> Goto1/1, CostFunctionofVoltageVectors/9(MPCC_f32DGridCurrentReference)
  MPCC_f32QGridCurrentReference/1 -> CostFunctionofVoltageVectors/10(MPCC_f32QGridCurrentReference)
  MPCC_f32DCLinkVoltage/1 -> Cast/1
  Gain/1 -> CostFunctionofVoltageVectors/11(MPCC_f32AlphaConvVoltage1)
  Gain1/1 -> CostFunctionofVoltageVectors/12(MPCC_f32AlphaConvVoltage2)
  Gain2/1 -> CostFunctionofVoltageVectors/13(MPCC_f32AlphaConvVoltage3)
  Gain3/1 -> CostFunctionofVoltageVectors/14(MPCC_f32AlphaConvVoltage4)
  Gain4/1 -> CostFunctionofVoltageVectors/15(MPCC_f32AlphaConvVoltage5)
  Gain5/1 -> CostFunctionofVoltageVectors/16(MPCC_f32AlphaConvVoltage6)
  Gain6/1 -> CostFunctionofVoltageVectors/17(MPCC_f32BetaConvVoltage1)
  Gain7/1 -> CostFunctionofVoltageVectors/18(MPCC_f32BetaConvVoltage2)
  Gain8/1 -> CostFunctionofVoltageVectors/19(MPCC_f32BetaConvVoltage3)
  Gain9/1 -> CostFunctionofVoltageVectors/20(MPCC_f32BetaConvVoltage4)
  Gain10/1 -> CostFunctionofVoltageVectors/21(MPCC_f32BetaConvVoltage5)
  Gain11/1 -> CostFunctionofVoltageVectors/22(MPCC_f32BetaConvVoltage6)
  [MPCC_f32CostFunction_Voltage1] -> CostFunctionofSectors/1(MPCC_f32CostFunction_Voltage1)
  [MPCC_f32CostFunction_Voltage4] -> CostFunctionofSectors/4(MPCC_f32CostFunction_Voltage4)
  [MPCC_f32CostFunction_Voltage5] -> CostFunctionofSectors/5(MPCC_f32CostFunction_Voltage5)
  [MPCC_f32CostFunction_Voltage6] -> CostFunctionofSectors/6(MPCC_f32CostFunction_Voltage6)
  [MPCC_f32CostFunction_Voltage2] -> CostFunctionofSectors/2(MPCC_f32CostFunction_Voltage2)
  [MPCC_f32CostFunction_Voltage3] -> CostFunctionofSectors/3(MPCC_f32CostFunction_Voltage3)
  CostFunctionofSectors/1(MPCC_f32CostFunction_Sector1) -> Mux/1
  CostFunctionofSectors/2(MPCC_f32CostFunction_Sector2) -> Mux/2
  CostFunctionofSectors/3(MPCC_f32CostFunction_Sector3) -> Mux/3
  CostFunctionofSectors/4(MPCC_f32CostFunction_Sector4) -> Mux/4
  CostFunctionofSectors/5(MPCC_f32CostFunction_Sector5) -> Mux/5
  CostFunctionofSectors/6(MPCC_f32CostFunction_Sector6) -> Mux/6
  Mux/1 -> Minimum/1
  MPCC_f32Duty_Sector1/1 -> CostFunctionofSectors/7(MPCC_f32Duty_Sector1)
  MPCC_f32Duty_Sector2/1 -> CostFunctionofSectors/8(MPCC_f32Duty_Sector2)
  MPCC_f32Duty_Sector3/1 -> CostFunctionofSectors/9(MPCC_f32Duty_Sector3)
  MPCC_f32Duty_Sector4/1 -> CostFunctionofSectors/10(MPCC_f32Duty_Sector4)
  MPCC_f32Duty_Sector5/1 -> CostFunctionofSectors/11(MPCC_f32Duty_Sector5)
  MPCC_f32Duty_Sector6/1 -> CostFunctionofSectors/12(MPCC_f32Duty_Sector6)
  Cast/1 -> Gain4/1, Gain9/1, Gain11/1, Gain10/1, Gain8/1, Gain7/1, Gain6/1, Gain5/1, Gain3/1, Gain/1, Gain1/1, Gain2/1
  Delay/1 -> [MPCC_f32CostFunction_Voltage1]
  Delay1/1 -> [MPCC_f32CostFunction_Voltage2]
  Delay2/1 -> [MPCC_f32CostFunction_Voltage3]
  Delay3/1 -> [MPCC_f32CostFunction_Voltage4]
  Delay4/1 -> [MPCC_f32CostFunction_Voltage5]
  Delay5/1 -> [MPCC_f32CostFunction_Voltage6]
  MPCC_f32QGridCurrent/1 -> CostFunctionofVoltageVectors/24(MPCC_f32QGridCurrent)
  MPCC_f32DGridCurrent/1 -> CostFunctionofVoltageVectors/23(MPCC_f32DGridCurrent)
  Minimum/1 -> MPCC_f32MinCostFunction/1
  Minimum/2 -> MPCC_f32MinSector/1
  MPCC_f32DGridCurrent1/1 -> CostFunctionofVoltageVectors/25(MPCC_f32DGridCurrent1)
  MPCC_f32QGridCurrent1/1 -> CostFunctionofVoltageVectors/26(MPCC_f32QGridCurrent1)

== system Copy_of_AB_Final_of_MPC_Bandwidth_Result/Subsystem1/ModulatorTimes ==
  MPCC_f32ElectricalAngle_K_1 : Inport
  MPCC_f32DCLinkVoltage : Inport  Port=2
  MPCC_f32Duty_Sector1 : Inport  Port=3
  MPCC_f32Duty_Sector2 : Inport  Port=4
  MPCC_f32Duty_Sector3 : Inport  Port=5
  MPCC_f32Duty_Sector4 : Inport  Port=6
  MPCC_f32Duty_Sector5 : Inport  Port=7
  MPCC_f32Duty_Sector6 : Inport  Port=8
  MPCC_f32MinSector : Inport  Port=9
  MPCC_f32SwitchingPeriod : Inport  Port=10
  Cast : DataTypeConversion  OutDataTypeStr=single  SaturateOnIntegerOverflow=off  RndMeth=Floor
  ConverterVoltage : Subsystem
  Gain : Gain  Gain=2/3
  Gain1 : Gain  Gain=1/3
  Gain10 : Gain  Gain=-1/sqrt(3)
  Gain11 : Gain  Gain=-1/sqrt(3)
  Gain2 : Gain  Gain=-1/3
  Gain3 : Gain  Gain=-2/3
  Gain4 : Gain  Gain=-1/3
  Gain5 : Gain  Gain=1/3
  Gain6 : Gain  Gain=0
  Gain7 : Gain  Gain=1/sqrt(3)
  Gain8 : Gain  Gain=1/sqrt(3)
  Gain9 : Gain  Gain=0
  ModulationVectorTimes : Subsystem
  MPCC_f32DQConvVoltage : Outport
  MPCC_f32Time1 : Outport  Port=2
  MPCC_f32Time2 : Outport  Port=3
  MPCC_f32Time0 : Outport  Port=4
  MPCC_u8ModulationSector : Outport  Port=5
  wires:
  MPCC_f32ElectricalAngle_K_1/1 -> ConverterVoltage/1(MPCC_f32ElectricalAngle_K_1)
  MPCC_f32DCLinkVoltage/1 -> Cast/1
  Gain/1 -> ConverterVoltage/2(MPCC_f32AlphaConvVoltage1)
  Gain1/1 -> ConverterVoltage/3(MPCC_f32AlphaConvVoltage2)
  Gain2/1 -> ConverterVoltage/4(MPCC_f32AlphaConvVoltage3)
  Gain3/1 -> ConverterVoltage/5(MPCC_f32AlphaConvVoltage4)
  Gain4/1 -> ConverterVoltage/6(MPCC_f32AlphaConvVoltage5)
  Gain5/1 -> ConverterVoltage/7(MPCC_f32AlphaConvVoltage6)
  Gain6/1 -> ConverterVoltage/8(MPCC_f32BetaConvVoltage1)
  Gain7/1 -> ConverterVoltage/9(MPCC_f32BetaConvVoltage2)
  Gain8/1 -> ConverterVoltage/10(MPCC_f32BetaConvVoltage3)
  Gain9/1 -> ConverterVoltage/11(MPCC_f32BetaConvVoltage4)
  Gain10/1 -> ConverterVoltage/12(MPCC_f32BetaConvVoltage5)
  Gain11/1 -> ConverterVoltage/13(MPCC_f32BetaConvVoltage6)
  ConverterVoltage/1(MPCC_f32DQConvVoltage) -> MPCC_f32DQConvVoltage/1
  MPCC_f32Duty_Sector5/1 -> [MPCC_f32Duty_Sector5]
  MPCC_f32Duty_Sector1/1 -> [MPCC_f32Duty_Sector1]
  MPCC_f32Duty_Sector6/1 -> [MPCC_f32Duty_Sector6]
  MPCC_f32Duty_Sector2/1 -> [MPCC_f32Duty_Sector2]
  MPCC_f32Duty_Sector4/1 -> [MPCC_f32Duty_Sector4]
  MPCC_f32Duty_Sector3/1 -> [MPCC_f32Duty_Sector3]
  MPCC_f32MinSector/1 -> [MPCC_f32MinSector], ConverterVoltage/20(MPCC_f32MinSector)
  [MPCC_f32Duty_Sector6] -> ConverterVoltage/19(MPCC_f32Duty_Sector6)
  [MPCC_f32Duty_Sector5] -> ConverterVoltage/18(MPCC_f32Duty_Sector5)
  [MPCC_f32Duty_Sector1] -> ConverterVoltage/14(MPCC_f32Duty_Sector1)
  [MPCC_f32Duty_Sector2] -> ConverterVoltage/15(MPCC_f32Duty_Sector2)
  [MPCC_f32Duty_Sector3] -> ConverterVoltage/16(MPCC_f32Duty_Sector3)
  [MPCC_f32Duty_Sector4] -> ConverterVoltage/17(MPCC_f32Duty_Sector4)
  [MPCC_f32Duty_Sector1] -> ModulationVectorTimes/1(MPCC_f32Duty_Sector1)
  [MPCC_f32Duty_Sector2] -> ModulationVectorTimes/2(MPCC_f32Duty_Sector2)
  [MPCC_f32Duty_Sector3] -> ModulationVectorTimes/3(MPCC_f32Duty_Sector3)
  [MPCC_f32Duty_Sector4] -> ModulationVectorTimes/4(MPCC_f32Duty_Sector4)
  [MPCC_f32Duty_Sector5] -> ModulationVectorTimes/5(MPCC_f32Duty_Sector5)
  [MPCC_f32Duty_Sector6] -> ModulationVectorTimes/6(MPCC_f32Duty_Sector6)
  MPCC_f32SwitchingPeriod/1 -> ModulationVectorTimes/7(MPCC_f32SwitchingPeriod)
  [MPCC_f32MinSector] -> ModulationVectorTimes/8(MPCC_f32MinSector)
  ModulationVectorTimes/3(MPCC_f32Time0) -> MPCC_f32Time0/1
  ModulationVectorTimes/1(MPCC_f32Time1) -> MPCC_f32Time1/1
  ModulationVectorTimes/2(MPCC_f32Time2) -> MPCC_f32Time2/1
  ModulationVectorTimes/4(MPCC_u8ModulationSector) -> MPCC_u8ModulationSector/1
  Cast/1 -> Gain/1, Gain4/1, Gain9/1, Gain11/1, Gain10/1, Gain8/1, Gain7/1, Gain6/1, Gain5/1, Gain3/1, Gain2/1, Gain1/1

== system Copy_of_AB_Final_of_MPC_Bandwidth_Result/Subsystem1/SOGI 1st ==
  w : Inport
  Vαβ : Inport  Port=2
  Gain : Gain  Gain=sqrt(2)  OutDataTypeStr=single
  Gain1 : Gain  Gain=0  OutDataTypeStr=single
  Integrator : Subsystem
  Integrator1 : Subsystem
  Integrator2 : Subsystem
  Multiply : Product
  Multiply1 : Product
  Multiply2 : Product
  Saturation : Saturate  UpperLimit=5  LowerLimit=-5
  Sum : Sum  Inputs=-+|
  Sum1 : Sum  Inputs=|+-
  Sum2 : Sum  Inputs=++|
  v : Outport
  qv : Outport  Port=2  OutDataTypeStr=single
  wires:
  w/1 -> Multiply2/2, Multiply/2, Multiply1/1
  Sum/1 -> Saturation/1, Gain/1
  Gain/1 -> Sum1/1
  Vαβ/1 -> Sum/2
  Sum1/1 -> Multiply/1
  Multiply/1 -> Integrator/1(In)
  Multiply2/1 -> Integrator2/1(In)
  Gain1/1 -> Multiply2/1
  Saturation/1 -> Gain1/1
  Integrator/1(Out) -> Sum2/2, v/1, Integrator1/1(In)
  Integrator1/1(Out) -> Multiply1/2
  Multiply1/1 -> Sum1/2, qv/1
  Integrator2/1(Out) -> Sum2/1
  Sum2/1 -> Sum/1

== system Copy_of_AB_Final_of_MPC_Bandwidth_Result/Subsystem1/SVM ==
  Vabc : Inport
  Vdc : Inport  Port=2
  Add : Sum
  Add1 : Sum
  Constant1 : Constant
  Divide : Product  Inputs=*/
  Gain : Gain  Gain=uint32(5000)
  Gain2 : Gain  Gain=0.5
  Gain8 : Gain  Gain=0.5
  Gain9 : Gain  Gain=0.5
  Max : MinMax  Function=max
  Max1 : MinMax
  Saturation : Saturate  UpperLimit=single(2/sqrt(3))  LowerLimit=single(-2/sqrt(3))
  Saturation1 : Saturate  UpperLimit=5000  LowerLimit=0
  Subtract : Sum  Inputs=+-
  Dabc : Outport
  wires:
  Max/1 -> Add/1
  Gain8/1 -> Divide/2
  Add1/1 -> Gain9/1
  Add/1 -> Gain2/1
  Vabc/1 -> Subtract/1, Max1/1, Max/1
  Max1/1 -> Add/2
  Divide/1 -> Saturation/1
  Constant1/1 -> Add1/2
  Gain2/1 -> Subtract/2
  Subtract/1 -> Divide/1
  Gain9/1 -> Gain/1
  Vdc/1 -> Gain8/1
  Saturation/1 -> Add1/1
  Gain/1 -> Saturation1/1
  Saturation1/1 -> Dabc/1

== system Copy_of_AB_Final_of_MPC_Bandwidth_Result/Subsystem1/Start ==
  Data : Inport
  Data_width : Inport  Port=2
  Action Port : ActionPort  ActionPortLabel=if(u1 == 0)
  Bias : Bias  Bias=1  SaturateOnIntegerOverflow=off
  End : Constant  Value=hex2dec('5353')  OutDataTypeStr=uint16
  Mux : Mux  Inputs=2
  Data_out : Outport  VectorParamsAs1DForOutWhenUnconnected=off
  Iteration : Outport  Port=2  VectorParamsAs1DForOutWhenUnconnected=off
  wires:
  End/1 -> Mux/1
  Mux/1 -> Data_out/1
  Data_width/1 -> Bias/1
  Bias/1 -> Iteration/1
  Data/1 -> Mux/2

== system Copy_of_AB_Final_of_MPC_Bandwidth_Result/Subsystem1/Start1 ==
  Data : Inport
  Data_width : Inport  Port=2
  Action Port : ActionPort  ActionPortLabel=if(u1 == 0)
  Bias : Bias  Bias=1  SaturateOnIntegerOverflow=off
  End : Constant  Value=hex2dec('5353')  OutDataTypeStr=uint16
  Mux : Mux  Inputs=2
  Data_out : Outport  VectorParamsAs1DForOutWhenUnconnected=off
  Iteration : Outport  Port=2  VectorParamsAs1DForOutWhenUnconnected=off
  wires:
  End/1 -> Mux/1
  Mux/1 -> Data_out/1
  Data_width/1 -> Bias/1
  Bias/1 -> Iteration/1
  Data/1 -> Mux/2
